simulink model "slcpp1"  (Simulink 6.3)
settings: Solver=ode45  SolverMode=SingleTasking  StartTime=0.0  StopTime=250  MaxStep=0.1  RelTol=1e-5  AbsTol=1e-6
PreLoadFcn:
  | initcpp1
undefined symbols (not defined in the file or in its folder): init_cond, pow, sgn
libraries: fuzblock x1
CloseFcn:
  | AnimFigTitle = [winName, ': Cart & Parallel Poles Animation']; AnimFigH = findobj(0,'Name',AnimFigTitle); close(AnimFigH)
settings Model: Creator=pascal  LastModifiedBy=mhaselti  ExtModeTrigMode=oneshot  ExtModeAutoUpdateStatusClock=off  StrictBusMsg=None
settings DataIOCC: LimitDataPoints=off  SaveOutput=off  SaveTime=off
settings OptimizationCC: BlockReduction=off  BooleanDataType=off
settings DebuggingCC: SolverPrmCheckMsg=none
settings HardwareCC: TargetUnknown=on
settings RTWCC: TemplateMakefile=grt_unix.tmf

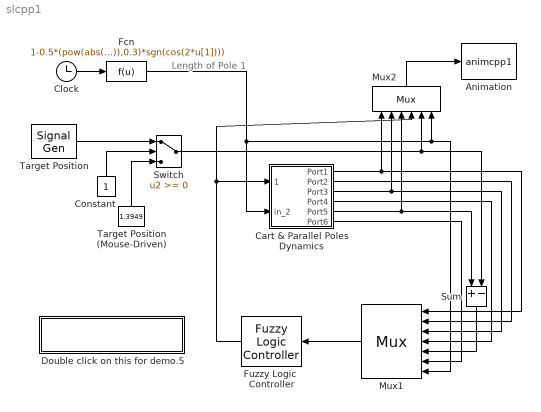
== system slcpp1 ==
  note: Length of Pole 1
  Animation : S-Function  FunctionName=animcpp1
  Cart & Parallel Poles Dynamics : Subsystem  mask(Differential Equation Editor (DEE)){init_cond =[-0.07 0 0.1 0 0 0],  specs =[1.0, 9.8]}
      mask prompts: init_cond  "Initial Conditions (a1, av1, a2, av2, x, v):";  specs  "Physical Specifications (M, g):"
      mask help: Inverted Pendulum (cart & two poles)
      mask init:
      | M=specs(1);g=specs(2);
      mask Display: plot(-4,-1,4,6,[0 3 2.8 -0.2 0]+0.5,[1 5 5.15 1.15 1],[0 0.2 -0.5 -0.7 0]-0.5, [1 1.2 2.7 2.5 1],[-1 -1 1 1 -1],[1 0 0 1 1],[-3.5 3.5],[0 0])
  Clock : Clock
      settings: Decimation=10
  Constant : Constant  Orientation=up
  Double click on this for demo.5 : Subsystem
      settings: OpenFcn=initcpp1
      mask Display: disp('Variable Initialization')
  Fcn : Fcn  Expr=1-0.5*(pow(abs(cos(2*u[1])),0.3)*sgn(cos(2*u[1])))
  Fuzzy Logic  Controller : fuzblock/Fuzzy Logic  Controller  Orientation=left  fis=fismat
  Mux1 : Mux  Orientation=left  Inputs=7
  Mux2 : Mux  Orientation=up  Inputs=6
  Sum : Sum  Orientation=down  Inputs=+-  SaturateOnIntegerOverflow=on  InputSameDT=on
  Switch : Switch  SaturateOnIntegerOverflow=on  InputSameDT=on
  Target Position : SignalGenerator  Amplitude=1.500000  Frequency=0.350000  Units=rad/sec
  Target Position (Mouse-Driven) : Constant  Orientation=up  Value=1.3949
  wires:
  Fcn/1 -> Mux1/7, Mux2/6, Cart & Parallel Poles Dynamics/2(in_2)
  Fuzzy Logic  Controller/1 -> Cart & Parallel Poles Dynamics/1(SysInport1), Mux2/4
  Clock/1 -> Fcn/1
  Target Position (Mouse-Driven)/1 -> Switch/3
  Constant/1 -> Switch/2
  Target Position/1 -> Switch/1
  Switch/1 -> Sum/2, Mux2/5
  Cart & Parallel Poles Dynamics/5(Port5) -> Sum/1, Mux2/3
  Sum/1 -> Mux1/5
  Mux2/1 -> Animation/1
  Cart & Parallel Poles Dynamics/3(Port3) -> Mux2/2, Mux1/3
  Cart & Parallel Poles Dynamics/1(Port1) -> Mux2/1, Mux1/1
  Cart & Parallel Poles Dynamics/6(Port6) -> Mux1/6
  Cart & Parallel Poles Dynamics/4(Port4) -> Mux1/4
  Cart & Parallel Poles Dynamics/2(Port2) -> Mux1/2
  Mux1/1 -> Fuzzy Logic  Controller/1

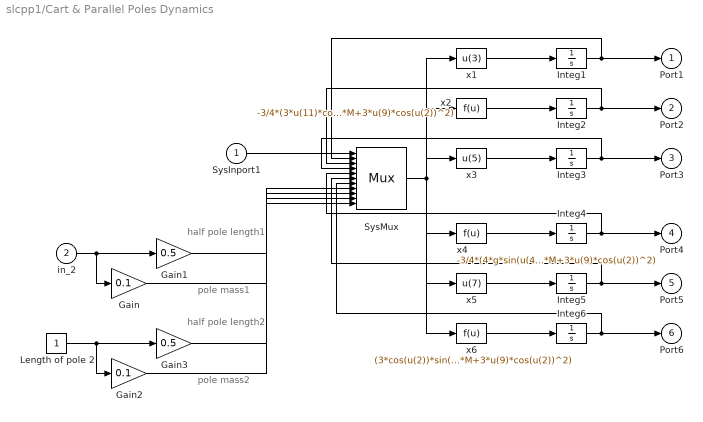
== system slcpp1/Cart & Parallel Poles Dynamics ==
  note: half pole length2
  note: pole mass2
  note: pole mass1
  note: half pole length1
  SysInport1 : Inport  Port=1  LatchInput=off
  in_2 : Inport  Port=2  LatchInput=off
  Gain : Gain  Gain=0.1  SaturateOnIntegerOverflow=on
  Gain1 : Gain  Gain=0.5  SaturateOnIntegerOverflow=on
  Gain2 : Gain  Gain=0.1  SaturateOnIntegerOverflow=on
  Gain3 : Gain  Gain=0.5  SaturateOnIntegerOverflow=on
  Integ1 : Integrator  InitialCondition=init_cond(1)
  Integ2 : Integrator  InitialCondition=init_cond(2)
  Integ3 : Integrator  InitialCondition=init_cond(3)
  Integ4 : Integrator  InitialCondition=init_cond(4)
  Integ5 : Integrator  InitialCondition=init_cond(5)
  Integ6 : Integrator  InitialCondition=init_cond(6)
  Length of pole 2 : Constant
  SysMux : Mux  Inputs=11
  x1 : Fcn  Expr=u(3)
  x2 : Fcn  Expr=-3/4*(3*u(11)*cos(u(4))*g*sin(u(4))*cos(u(2))-4*u(11)*u(10)*sin(u(4))*u(5)^2*cos(u(2))+4*sin(u(2))*g*M+4*sin(u(2))*g*u(9)+4*sin(u(2))*g*u(11)-3*sin(u(2))*g*u(11)*cos(u(4))^2-4*u(1)*cos(u(2))-4*u(9)*u(8)*sin(u(2))*u(3)^2*cos(u(2)))/u(8)/(3*u(11)*cos(u(4))^2-4*u(9)-4*u(11)-4*M+3*u(9)*cos(u(2))^2)
  x3 : Fcn  Expr=u(5)
  x4 : Fcn  Expr=-3/4*(4*g*sin(u(4))*u(9)+4*g*sin(u(4))*u(11)-4*u(11)*u(10)*sin(u(4))*u(5)^2*cos(u(4))+4*g*sin(u(4))*M-3*g*sin(u(4))*u(9)*cos(u(2))^2+3*cos(u(4))*cos(u(2))*sin(u(2))*g*u(9)-4*cos(u(4))*u(1)-4*cos(u(4))*u(9)*u(8)*sin(u(2))*u(3)^2)/u(10)/(3*u(11)*cos(u(4))^2-4*u(9)-4*u(11)-4*M+3*u(9)*cos(u(2))^2)
  x5 : Fcn  Expr=u(7)
  x6 : Fcn  Expr=(3*cos(u(2))*sin(u(2))*g*u(9)+3*u(11)*cos(u(4))*g*sin(u(4))-4*u(1)-4*u(9)*u(8)*sin(u(2))*u(3)^2-4*u(11)*u(10)*sin(u(4))*u(5)^2)/(3*u(11)*cos(u(4))^2-4*u(9)-4*u(11)-4*M+3*u(9)*cos(u(2))^2)
  Port1 : Outport  InitialOutput=0
  Port2 : Outport  Port=2  InitialOutput=0
  Port3 : Outport  Port=3  InitialOutput=0
  Port4 : Outport  Port=4  InitialOutput=0
  Port5 : Outport  Port=5  InitialOutput=0
  Port6 : Outport  Port=6  InitialOutput=0
  wires:
  Integ6/1 -> Port6/1, SysMux/7
  Integ5/1 -> Port5/1, SysMux/6
  Integ4/1 -> Port4/1, SysMux/5
  Integ3/1 -> Port3/1, SysMux/4
  Integ2/1 -> Port2/1, SysMux/3
  Integ1/1 -> Port1/1, SysMux/2
  SysInport1/1 -> SysMux/1
  x1/1 -> Integ1/1
  x2/1 -> Integ2/1
  x3/1 -> Integ3/1
  x4/1 -> Integ4/1
  SysMux/1 -> x1/1, x2/1, x3/1, x4/1, x5/1, x6/1
  x5/1 -> Integ5/1
  x6/1 -> Integ6/1
  Gain3/1 -> SysMux/10
  Length of pole 2/1 -> Gain3/1, Gain2/1
  Gain2/1 -> SysMux/11
  Gain/1 -> SysMux/9
  in_2/1 -> Gain1/1, Gain/1
  Gain1/1 -> SysMux/8

== system slcpp1/Double click on this for demo.5 ==
